simulink model "haptic_device_speed_limit_MODEL"  (R2020a)
settings: Solver=VariableStepAuto  StartTime=0.0  StopTime=16  RelTol=1e-3
libraries: simulink x1
settings Model: Creator=Lotnik  LastModifiedBy=Lotnik

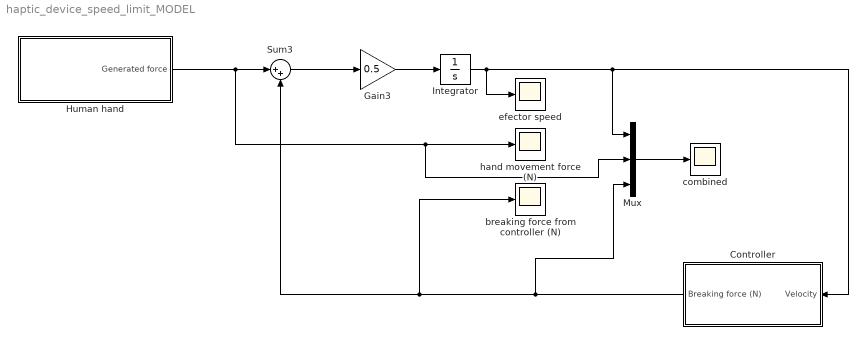
== system haptic_device_speed_limit_MODEL ==
  Controller : Subsystem
  Gain3 : Gain  Gain=0.5
  Human hand : Subsystem
  Integrator : Integrator
  Mux : Mux  Inputs=3
  Sum3 : Sum  Inputs=|++
  breaking force from controller (N) : Scope
  combined : Scope
  efector speed : Scope
  hand movement force (N) : Scope
  wires:
  Sum3/1 -> Gain3/1
  Gain3/1 -> Integrator/1
  Integrator/1 -> Controller/1(Velocity), Mux/1, efector speed/1
  Mux/1 -> combined/1
  Human hand/1(Generated force) -> hand movement force (N)/1, Mux/2, Sum3/1
  Controller/1(Breaking force (N)) -> Mux/3, breaking force from controller (N)/1, Sum3/2

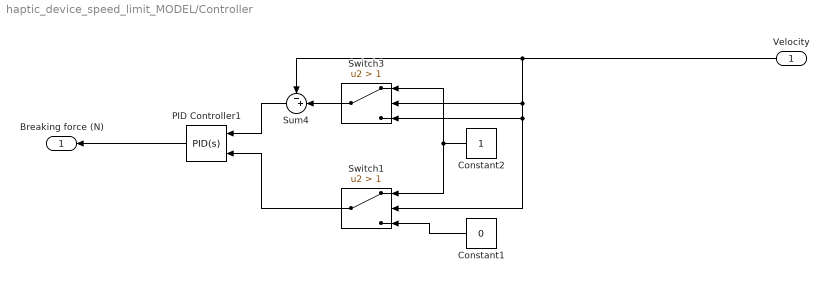
== system haptic_device_speed_limit_MODEL/Controller ==
  Velocity : Inport
  Constant1 : Constant  Value=0
  Constant2 : Constant
  PID Controller1 : simulink/Continuous/PID Controller  Controller=PID  Form=Parallel  TimeDomain=Continuous-time  UseExternalTs=off  SampleTime=-1  IntegratorMethod=Forward Euler  FilterMethod=Forward Euler  ControllerParametersSource=internal  P=30  I=4  D=0  UseFilter=on  N=100  TunerSelectOption=Transfer Function Based (PID Tuner App)  InitialConditionSource=internal  InitialConditionForIntegrator=0  InitialConditionForFilter=0  DifferentiatorICPrevScaledInput=0  ExternalReset=falling  TrackingMode=off  Kt=1  LimitOutput=off  UpperSaturationLimit=inf  LowerSaturationLimit=-inf  LinearizeAsGain=on  AntiWindupMode=none  Kb=1  POutMin=[]  POutMax=[]  IOutMin=[]  IOutMax=[]  DOutMin=[]  DOutMax=[]  NOutMin=[]  NOutMax=[]  SumOutMin=[]  SumOutMax=[]  SaturationOutMin=[]  SaturationOutMax=[]  PParamMin=[]  PParamMax=[]  IParamMin=[]  IParamMax=[]  DParamMin=[]  DParamMax=[]  NParamMin=[]  NParamMax=[]  KbParamMin=[]  KbParamMax=[]  KtParamMin=[]  KtParamMax=[]  KbOutMin=[]  KbOutMax=[]  KtOutMin=[]  KtOutMax=[]  IntegratorOutMin=[]  IntegratorOutMax=[]  FilterOutMin=[]  FilterOutMax=[]  SumI1OutMin=[]  SumI1OutMax=[]  SumI2OutMin=[]  SumI2OutMax=[]  SumI3OutMin=[]  SumI3OutMax=[]  SumI4OutMin=[]  SumI4OutMax=[]  SumDOutMin=[]  SumDOutMax=[]  DifferentiatorOutMin=[]  DifferentiatorOutMax=[]  FilterDiffOutCoefMin=[]  FilterDiffOutCoefMax=[]  ReciprocalOutMin=[]  ReciprocalOutMax=[]  SumDenOutMin=[]  SumDenOutMax=[]  SumNumOutMin=[]  SumNumOutMax=[]  DivideOutMin=[]  DivideOutMax=[]  UdiffTsProdOutMin=[]  UdiffTsProdOutMax=[]  NTsProdOutMin=[]  NTsProdOutMax=[]  UintegralTsProdOutMin=[]  UintegralTsProdOutMax=[]  UngainTsProdOutMin=[]  UngainTsProdOutMax=[]  IntegratorContinuousStateAttributes=''  IntegratorStateMustResolveToSignalObject=off  IntegratorRTWStateStorageClass=Auto  FilterContinuousStateAttributes=''  FilterStateMustResolveToSignalObject=off  FilterRTWStateStorageClass=Auto  ParallelPVariant=InternalParameters  IdealPVariant=Disabled  IVariant=InternalParameters  DVariant=InternalParameters  IntegratorVariant=Continuous  SatVariant=Disabled  AWVariant=Passthrough  PCopyVariant=Disabled  TRVariant=Disabled  FdbkBlocksVariant=Forward  IdealPFdbkVariant=Disabled  SatFdbkVariant=Disabled  DerivativeFilterVariant=ContFilter  NVariant=InternalParameters  NCopyVariant=Disabled  FilterICVariant=InternalICsFilter  IntegratorICVariant=InternalICs  ExternalResetVariant=ExternalReset  TRSumVariant=Passthrough  SumFdbkVariant=Disabled  SumVariant=Sum_PID  TsampFilterVariant=InternalTs  TsampNgainVariant=Passthrough  TsampIntegralVariant=Passthrough
  Sum4 : Sum  Inputs=-+|
  Switch1 : Switch  Criteria=u2 > Threshold  Threshold=1
  Switch3 : Switch  Criteria=u2 > Threshold  Threshold=1
  Breaking force (N) : Outport
  wires:
  Switch3/1 -> Sum4/2
  Constant2/1 -> Switch3/1, Switch1/1
  PID Controller1/1 -> Breaking force (N)/1
  Velocity/1 -> Sum4/1, Switch3/2, Switch3/3, Switch1/2
  Sum4/1 -> PID Controller1/1
  Switch1/1 -> PID Controller1/2
  Constant1/1 -> Switch1/3

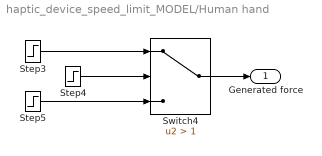
== system haptic_device_speed_limit_MODEL/Human hand ==
  Step3 : Step  Time=10  Before=3  After=0  SampleTime=0
  Step4 : Step  Time=4  After=2  SampleTime=0
  Step5 : Step  Time=2  Before=2  After=0  SampleTime=0
  Switch4 : Switch  Criteria=u2 > Threshold  Threshold=1
  Generated force : Outport
  wires:
  Step3/1 -> Switch4/1
  Step5/1 -> Switch4/3
  Step4/1 -> Switch4/2
  Switch4/1 -> Generated force/1
